simulink model "closeloop2PIBCR2023a"  (R2023a)
settings: Solver=ode1  StartTime=0.0  StopTime=1  FixedStep=1e-6  MaxStep=1e-6  RelTol=1e-3
PreLoadFcn:
  | L=32e-6;
  | k=-1/3;
  | M=  L*k
  | %N=4 %nbre de spires
  | rL=3.34e-3;
  | V_dc=14.4;
  | C=100e-6;
  | r_load=5;
undefined symbols (not defined in the file): plecs, sigbuilder_block
libraries: eePwmGenerator x2
settings Model: Creator=QUDUS  LastModifiedBy=QUDUS
settings SolverCC: ZeroCrossAlgorithm=Adaptive
settings DebuggingCC: IgnoredZcDiagnostic=none
settings RTWCC: GPUComputeCapability=5.0

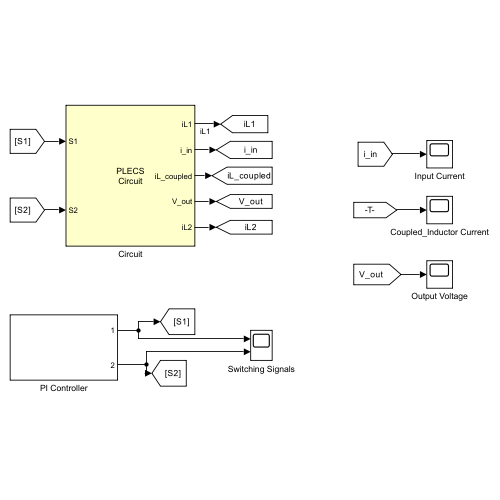
[thumbnail: Simulink's stored preview of the top-level diagram]
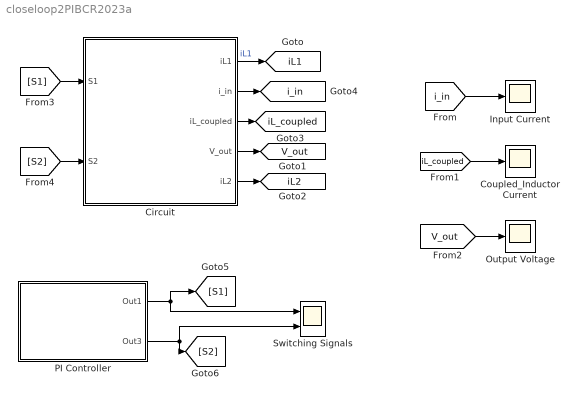
== system closeloop2PIBCR2023a ==
  Circuit : Subsystem  LoadFcn=plecs('sl', 200);  InitFcn=plecs('sl', 214);  StartFcn=plecs('sl', 208);  StopFcn=plecs('sl', 209);  ClipboardFcn=plecs('sl', 212, 13);  mask(PlecsCircuit){PLECSData=<binary blob, 3964 chars, not shown>}
      mask prompts: PLECSData "PLECS Data (Do not delete or modify!)"
      mask init:
      | % PLACE CUSTOM INITIALIZATIONS ABOVE
      | % DO NOT REMOVE
      | plecs('sl', 215);
      | % DO NOT REMOVE
      settings: CopyFcn=plecs('sl', 203);  DeleteFcn=plecs('sl', 205);  UndoDeleteFcn=plecs('sl', 206);  PreSaveFcn=plecs('sl', 211);  PostSaveFcn=plecs('sl', 201);  NameChangeFcn=plecs('sl', 210);  DestroyFcn=plecs('sl', 207);  PreCopyFcn=plecs('sl', 216);  OpenFcn=plecs('sl', 202);  ErrorFcn=plerrorfcn
      mask Help: eval('plecs(''help'', ''qthelp:///creatingacircuit.html'')')
      mask Display: disp('PLECS\nCircuit')
  Coupled_Inductor Current : Scope
  Input Current : Scope
  Output Voltage : Scope
  PI Controller : Subsystem
  Switching Signals : Scope  NumInputPorts=2
  tag scope: V_out=global, iL1=global, iL2=global, iL_coupled=global, i_in=global
  wires:
  Circuit/3(iL_coupled) -> [iL_coupled]
  Circuit/2(i_in) -> [i_in]
  Circuit/4(V_out) -> [V_out]
  Circuit/5(iL2) -> [iL2]
  [S2] -> Circuit/2(S2)
  [S1] -> Circuit/1(S1)
  Circuit/1(iL1) -> [iL1]  "iL1"
  [i_in] -> Input Current/1
  [iL_coupled] -> Coupled_Inductor Current/1
  [V_out] -> Output Voltage/1
  PI Controller/2(Out3) -> Switching Signals/2, [S2]
  PI Controller/1(Out1) -> [S1], Switching Signals/1

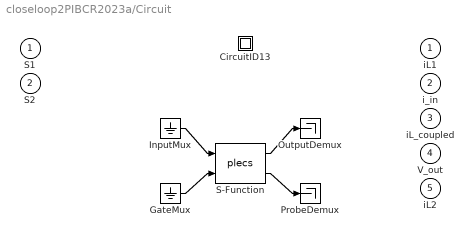
== system closeloop2PIBCR2023a/Circuit ==
  S1 : Inport  PortDimensions=1
  S2 : Inport  Port=2  PortDimensions=1
  " CircuitID13 " : Subsystem
  " GateMux " : Ground
  " InputMux " : Ground
  " OutputDemux " : Terminator
  " ProbeDemux " : Terminator
  " S-Function " : S-Function  FunctionName=plecs  SFunctionDeploymentMode=off  EnableBusSupport=off
  iL1 : Outport  PortDimensions=1
  i_in : Outport  Port=2  PortDimensions=1
  iL_coupled : Outport  Port=3  PortDimensions=2
  V_out : Outport  Port=4  PortDimensions=1
  iL2 : Outport  Port=5  PortDimensions=1
  wires:
  " InputMux "/1 -> " S-Function "/1
  " GateMux "/1 -> " S-Function "/2
  " S-Function "/1 -> " OutputDemux "/1
  " S-Function "/2 -> " ProbeDemux "/1

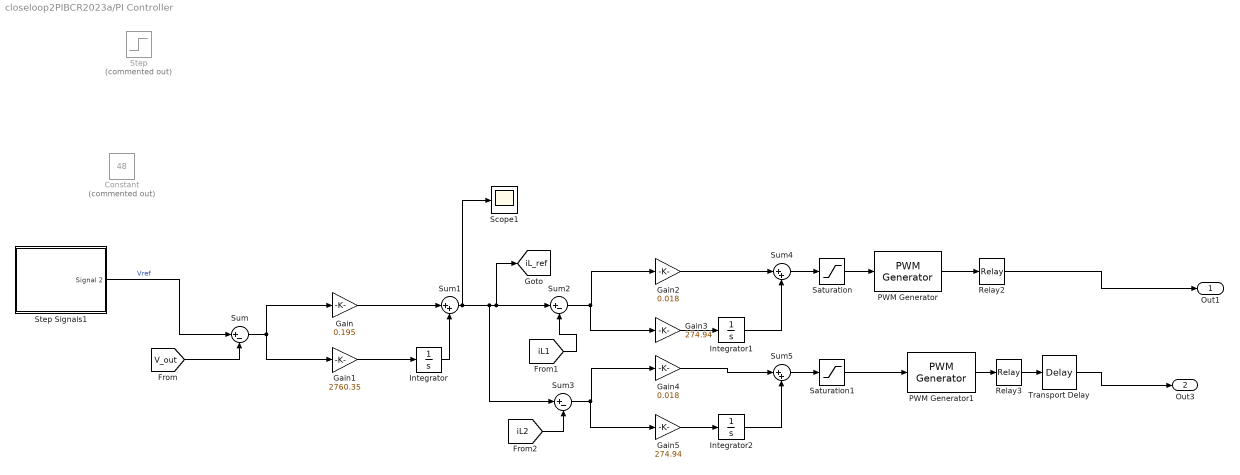
== system closeloop2PIBCR2023a/PI Controller ==
  Constant : Constant  Commented=on  Value=48
  Gain : Gain  Gain=0.195
  Gain1 : Gain  Gain=2760.35
  Gain2 : Gain  Gain=0.018
  Gain3 : Gain  Gain=274.94
  Gain4 : Gain  Gain=0.018
  Gain5 : Gain  Gain=274.94
  Integrator : Integrator
  Integrator1 : Integrator
  Integrator2 : Integrator
  PWM Generator : eePwmGenerator/PWM Generator  CarrCount=Up  Tper=2e-5  Tdelay=0  Ts=0
  PWM Generator1 : eePwmGenerator/PWM Generator  CarrCount=Up  Tper=2e-5  Tdelay=0  Ts=0
  Relay2 : Relay
  Relay3 : Relay
  Saturation : Saturate  UpperLimit=0.9  LowerLimit=0.1
  Saturation1 : Saturate  UpperLimit=0.9  LowerLimit=0.1
  Scope1 : Scope
  Step : Step  Commented=on  Time=0.06  Before=48  After=40  SampleTime=0
  Step Signals1 : Subsystem  Tag=STV Subsys  LoadFcn=sigbuilder_block('load');  StartFcn=sigbuilder_block('start');  StopFcn=sigbuilder_block('stop');  ClipboardFcn=sigbuilder_block('clipboard');  mask(Sigbuilder block){tuvar=[0:10]}
      mask help: Simulink:masks:SigbuilderBlock_MD
      mask init:
      | if ~strcmp(get_param(bdroot(gcbh),'SimulationStatus'),'stopped') tuvar = sigbuilder_block('maskInit'); end
      settings: CopyFcn=sigbuilder_block('copy');  DeleteFcn=sigbuilder_block('delete');  ModelCloseFcn=sigbuilder_block('modelClose');  PreSaveFcn=sigbuilder_block('preSave');  PauseFcn=sigbuilder_block('pause');  ContinueFcn=sigbuilder_block('continue');  NameChangeFcn=sigbuilder_block('namechange');  OpenFcn=sigbuilder_block('open',[6 36 1428 675.75 ]);  CloseFcn=sigbuilder_block('close');
      mask Display: plot(0, 0, 100, 100,[2, 2, 32, 32, 2], [68, 8, 8, 68, 68],[32, 2], [38, 38], [32, 19, 2],[53, 60, 44], [32, 17, 17, 2],[16, 16, 31, 31]);txt = getActiveGroup(gcbh);text(2, 100, txt,'verticalAlignment', 'top');
  Sum : Sum  Inputs=|+-
  Sum1 : Sum  Inputs=|++
  Sum2 : Sum  Inputs=|+-
  Sum3 : Sum  Inputs=|+-
  Sum4 : Sum  Inputs=|++
  Sum5 : Sum  Inputs=|++
  Transport Delay : TransportDelay  DelayTime=1e-5
  Out1 : Outport
  Out3 : Outport  Port=2
  tag scope: iL_ref=global
  wires:
  [V_out] -> Sum/2
  Gain5/1 -> Integrator2/1
  Sum1/1 -> Sum3/1, Sum2/1, [iL_ref], Scope1/1
  Gain4/1 -> Sum5/1
  Gain2/1 -> Sum4/1
  Sum3/1 -> Gain5/1, Gain4/1
  Integrator1/1 -> Sum4/2
  Relay3/1 -> Transport Delay/1
  Integrator2/1 -> Sum5/2
  Transport Delay/1 -> Out3/1
  [iL1] -> Sum2/2
  Gain1/1 -> Integrator/1
  [iL2] -> Sum3/2
  Sum/1 -> Gain1/1, Gain/1
  PWM Generator/1 -> Relay2/1
  Sum2/1 -> Gain3/1, Gain2/1
  Integrator/1 -> Sum1/2
  Saturation/1 -> PWM Generator/1
  Gain/1 -> Sum1/1
  Gain3/1 -> Integrator1/1
  Sum5/1 -> Saturation1/1
  Sum4/1 -> Saturation/1
  PWM Generator1/1 -> Relay3/1
  Saturation1/1 -> PWM Generator1/1
  Relay2/1 -> Out1/1
  Step Signals1/1(Signal 2) -> Sum/1  "Vref"

== system closeloop2PIBCR2023a/Circuit/ CircuitID13  ==

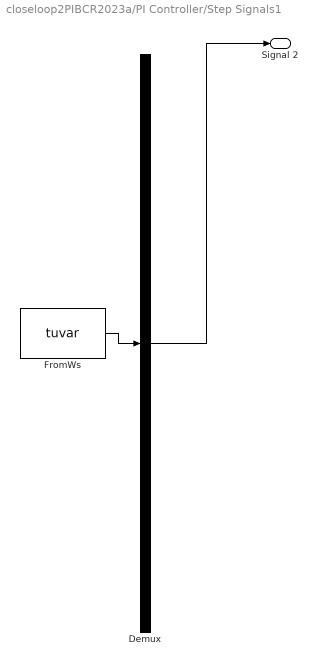
== system closeloop2PIBCR2023a/PI Controller/Step Signals1 ==
  Demux : Demux  Tag=STV Demux  Outputs=1
      settings: DisplayOption=none
  FromWs : FromWorkspace  Tag=STV FromWs  VariableName=tuvar
      SigBuilderData=|
      | common.afterFinalStr = 'Extrapolate'
      | common.sampleTime = 0
      | dataSet.timeRange = [0 35]
      | dataSet.name = 'Group 1'
      | sbobj.Groups.Name = 'Group 1'
      | sbobj.Groups.Signals.Name = 'Signal 2'
      | sbobj.Groups.Signals.XData = [0 0.01 0.2 0.2 0.4 0.4 0.6 0.6 0.801 0.801 1.01 1.01 20.001 20.001 25 25 35]
      | sbobj.Groups.Signals.YData = [60 60 60 48.5 48.5 40 40 30 30 48 47.5 0 84 122 122 98.5 97]
      | sbobj.Groups.TimeRange = [0 35]
  Signal 2 : Outport  Tag=STV Outport
  wires:
  Demux/1 -> Signal 2/1
  FromWs/1 -> Demux/1
